simulink model "Subsystems"  (R2024b)
settings: Solver=VariableStepAuto  StartTime=0.0  StopTime=10.0  RelTol=1e-3
undefined symbols (not defined in the file): AirSpeed, Gravity, Height, RollAngle, WindDown, WindEast, WindNorth
libraries: uavalgslib x1

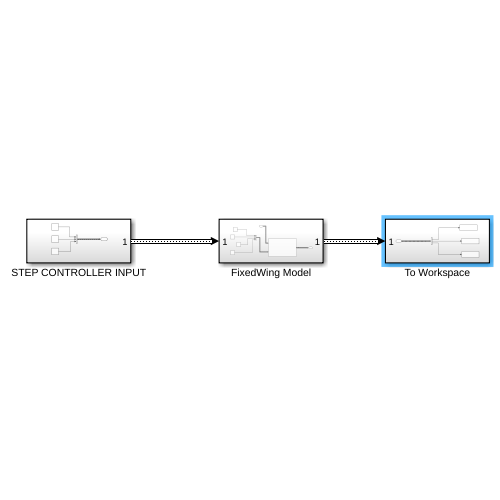
[thumbnail: Simulink's stored preview of the top-level diagram]
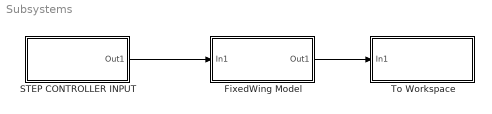
== system Subsystems ==
  FixedWing Model : Subsystem
  STEP CONTROLLER INPUT : Subsystem
  To Workspace : Subsystem
  wires:
  STEP CONTROLLER INPUT/1(Out1) -> FixedWing Model/1(In1)
  FixedWing Model/1(Out1) -> To Workspace/1(In1)

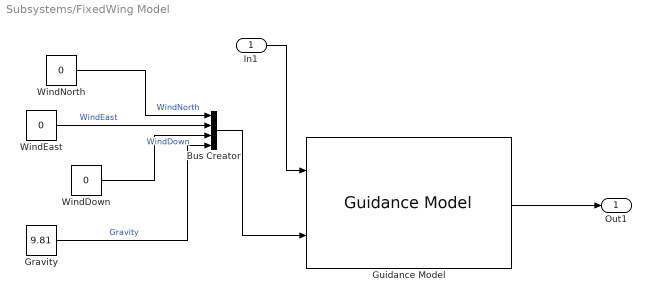
== system Subsystems/FixedWing Model ==
  In1 : Inport
  Bus Creator : BusCreator  Inputs=WindNorth,WindEast,WindDown,Gravity  OutDataTypeStr=Bus: FixedWingGuidanceEnvironmentBus  NonVirtualBus=on
  Gravity : Constant  Value=9.81
  Guidance Model : uavalgslib/Guidance Model  ModelType=FixedWingGuidance  SpecifiedDataType=double  SimulateUsing=Interpreted execution  InitialWorldPositionMultirotor=[0; 0; 0]  InitialWorldVelocityMultirotor=[0; 0; 0]  InitialEulerZYXMultirotor=[0; 0; 0]  InitialBodyAngularRateRPYMultirotor=[0; 0; 0]  InitialThrustMultirotor=0  InitialNorthFixedWing=0  InitialEastFixedWing=0  InitialHeightFixedWing=0  InitialAirSpeedFixedWing=0  InitialHeadingAngleFixedWing=0  InitialFlightPathAngleFixedWing=0  InitialRollAngleFixedWing=0  InitialRollAngleRateFixedWing=0  PDRollMultirotor=[3402.97,116.67]  PDPitchMultirotor=[3402.97, 116.67]  PYawRateMultirotor=1950  PThrustMultirotor=3900  MassMultirotor=0.1  PHeightFixedWing=3.9  PHeadingAngleFixedWing=3.9  PFlightPathAngleFixedWing=39  PDRollFixedWing=[3402.97, 116.67]  PAirSpeedFixedWing=1  FlightPathAngleLimitsFixedWing=[-pi/2, pi/2]  StateBusName='FixedWingGuidanceStateBus'  ControlBusName='FixedWingGuidanceControlBus'  EnvironmentBusName='FixedWingGuidanceEnvironmentBus'  DataType=double
  WindDown : Constant  Value=0
  WindEast : Constant  Value=0
  WindNorth : Constant  Value=0
  Out1 : Outport
  wires:
  Bus Creator/1 -> Guidance Model/2
  Gravity/1 -> Bus Creator/4  "Gravity"
  WindDown/1 -> Bus Creator/3  "WindDown"
  WindNorth/1 -> Bus Creator/1  "WindNorth"
  WindEast/1 -> Bus Creator/2  "WindEast"
  In1/1 -> Guidance Model/1
  Guidance Model/1 -> Out1/1

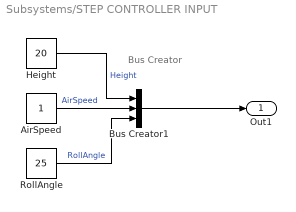
== system Subsystems/STEP CONTROLLER INPUT ==
  note: Bus Creator
  AirSpeed : Constant
  Bus Creator1 : BusCreator  Inputs=Height,AirSpeed,RollAngle  OutDataTypeStr=Bus: FixedWingGuidanceControlBus  NonVirtualBus=on
  Height : Constant  Value=20
  RollAngle : Constant  Value=25
  Out1 : Outport
  wires:
  Height/1 -> Bus Creator1/1  "Height"
  RollAngle/1 -> Bus Creator1/3  "RollAngle"
  AirSpeed/1 -> Bus Creator1/2  "AirSpeed"
  Bus Creator1/1 -> Out1/1

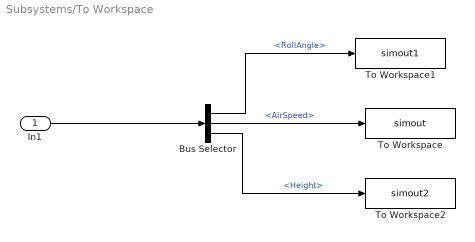
== system Subsystems/To Workspace ==
  In1 : Inport
  Bus Selector : BusSelector  OutputSignals=RollAngle,AirSpeed,Height
  To Workspace : ToWorkspace  VariableName=simout  SaveFormat=Timeseries  SampleTime=-1
  To Workspace1 : ToWorkspace  VariableName=simout1  SaveFormat=Timeseries  SampleTime=-1
  To Workspace2 : ToWorkspace  VariableName=simout2  SaveFormat=Timeseries  SampleTime=-1
  wires:
  Bus Selector/3 -> To Workspace2/1  "<Height>"
  Bus Selector/2 -> To Workspace/1  "<AirSpeed>"
  Bus Selector/1 -> To Workspace1/1  "<RollAngle>"
  In1/1 -> Bus Selector/1
